simulink model "Tekercs_H6"  (R2025a)
settings: Solver=VariableStepAuto  StartTime=0.0  StopTime=50e-3  MaxStep=1e-3/25  RelTol=1e-3
settings Model: Creator=Szalay  LastModifiedBy=Szalay

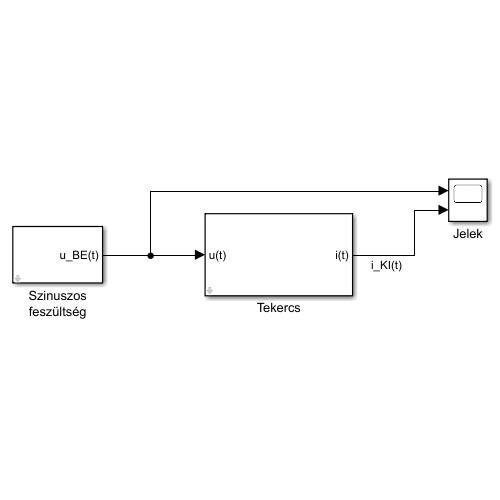
[thumbnail: Simulink's stored preview of the top-level diagram]
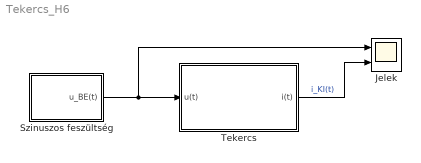
== system Tekercs_H6 ==
  Jelek : Scope  NumInputPorts=2
      settings: ActiveDisplayYMinimum=-1.2498696653726216  ActiveDisplayYMaximum=1.2499855183747357
  Szinuszos feszültség : Subsystem  mask(Szinuszos feszültség){A=1, f=1000/(2*pi), q=0}
      mask prompts: A "Amplitúdó"; f "Frekvencia (Hz)"; q "Fáziseltolódás (rad)"
      mask help: Paraméterezhető szinuszos feszültségforrás u_BE(t) = A cos(2 π f t + φ) alakban.
      mask DialogControl ParameterGroupVar Prompt: Beállítások
  Tekercs : Subsystem  mask(Tekercsmodell){R=2, L=2e-3, i_0=0.5}
      mask prompts: R "Ellenállás (Ohm)"; L "Öninduktivitás (H)"; i_0 "Az áramerősség kezdeti értéke (A)"
      mask help: Lineáris mágnesezettségű tekercs (RL-tag) modellje.
      mask DialogControl ParameterGroupVar Prompt: Modellparaméterek
      mask DialogControl Container3 Prompt: Kezdeti érték
  wires:
  Tekercs/1(i(t)) -> Jelek/2  "i_KI(t)"
  Szinuszos feszültség/1(u_BE(t)) -> Jelek/1, Tekercs/1(u(t))

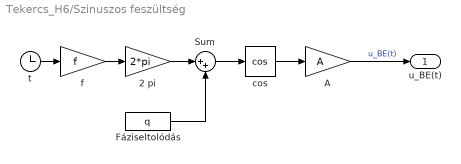
== system Tekercs_H6/Szinuszos feszültség ==
  2 pi : Gain  Gain=2*pi
  A : Gain  Gain=A
  Fáziseltolódás : Constant  Value=q
  Sum : Sum  Inputs=|++
  cos : Trigonometry  Operator=cos
  f : Gain  Gain=f
  t : Clock
  u_BE(t) : Outport
  wires:
  t/1 -> f/1
  f/1 -> 2 pi/1
  2 pi/1 -> Sum/1
  A/1 -> u_BE(t)/1  "u_BE(t)"
  cos/1 -> A/1
  Sum/1 -> cos/1
  Fáziseltolódás/1 -> Sum/2

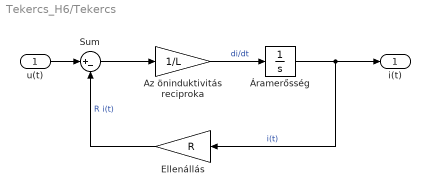
== system Tekercs_H6/Tekercs ==
  u(t) : Inport
  Az öninduktivitás reciproka : Gain  Gain=1/L
  Ellenállás : Gain  Gain=R
  Sum : Sum  Inputs=|+-
  Áramerősség : Integrator  InitialCondition=i_0
  i(t) : Outport
  wires:
  Az öninduktivitás reciproka/1 -> Áramerősség/1  "di/dt"
  u(t)/1 -> Sum/1
  Áramerősség/1 -> i(t)/1, Ellenállás/1  "i(t)"
  Ellenállás/1 -> Sum/2  "R i(t)"
  Sum/1 -> Az öninduktivitás reciproka/1
